simulink model "Model_5"  (R2020b)
settings: Solver=VariableStepAuto  StartTime=0.0  StopTime=10.0  RelTol=1e-3
values from neighbouring files (symbols this model uses):
  C = 25    [Problem_5.mat]    (also in Variables.m = 0.5)
  R = 15    [Problem_5.mat]    (also in Variables.m = 5)
settings Model: Creator=samar  LastModifiedBy=samar

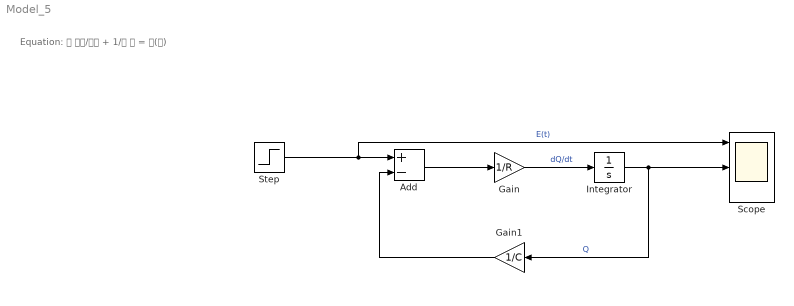
== system Model_5 ==
  note: Equation:
      | 𝑅 𝑑𝑄/𝑑𝑡 + 1/𝐶 𝑄 = 𝐸(𝑡)
  Add : Sum  Inputs=+-
  Gain : Gain  Gain=1/R
  Gain1 : Gain  Gain=1/C
  Integrator : Integrator
  Scope : Scope  NumInputPorts=3
  Step : Step  SampleTime=0
  wires:
  Step/1 -> Scope/1, Add/1  "E(t)"
  Add/1 -> Gain/1
  Gain/1 -> Integrator/1  "dQ/dt"
  Integrator/1 -> Gain1/1, Scope/2  "Q"
  Gain1/1 -> Add/2
